simulink model "rx_chain_blockset"  (R2022b)
settings: Solver=VariableStepAuto  StartTime=0.0  StopTime=0  RelTol=1e-3
undefined symbols (not defined in the file or in its folder): rf, S
libraries: simrfV2elements x7, simrfV2util1 x4, rfBudgetAnalyzer_lib x3, simrfV2systems x2, simrfV2sources1 x1
settings Model: Creator=hessam  LastModifiedBy=hessam

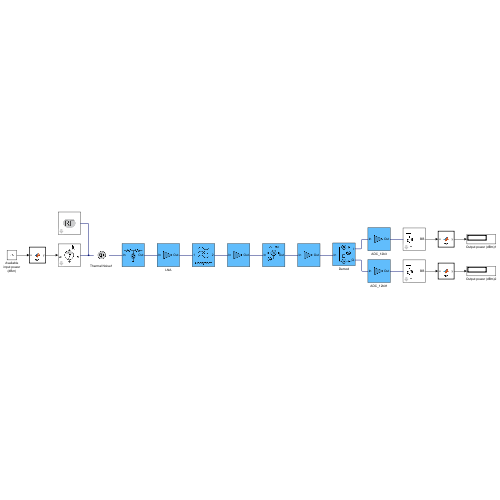
[thumbnail: Simulink's stored preview of the top-level diagram]
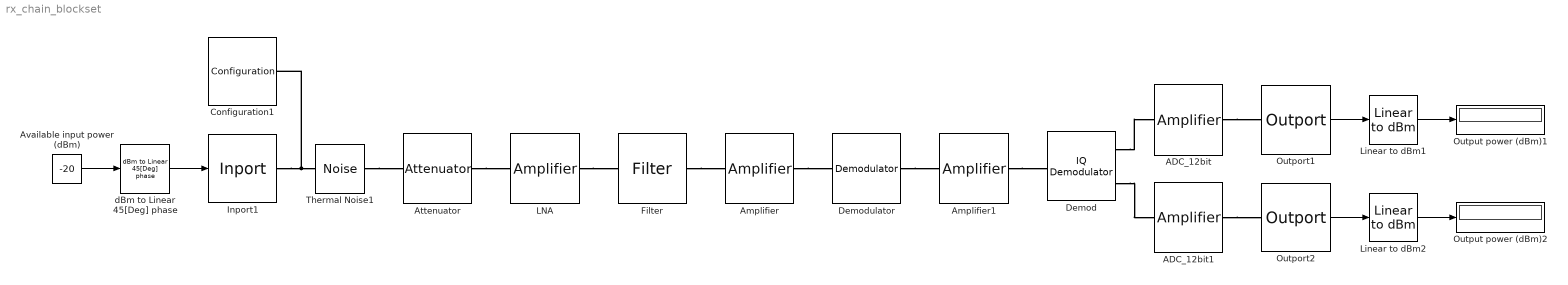
== system rx_chain_blockset ==
  ADC_12bit : simrfV2elements/Amplifier  classname=amplifier  DataSource=Data file  isNetworkObj=off  Paramtype=S-parameters  Sparam=[0 0;1 0]  SparamFreq=1e9 Hz  SparamZ0=50  isRationalObj=off  Residues=0  Poles=0  DF={0 0; 1 0}  Source_linear_gain=Available power gain  linear_gain=0 dB  AmAmAmPmTable=[-25,5,-1;-10,20,-2;0,27,5;5,28,12]  Zin=50  Zout=50  Source_Poly=Even and odd order  Poly_Coeffs=[0 1]  IPType=Output  IP2=Inf dBm  IP3=Inf dBm  P1dB=inf dBm  Psat=inf dBm  Gcomp=inf dBm  InternalGrounding=on  SourceFreq=Extracted from data source  PlotFreq=[1e9:1e6:3e9] Hz  PlotType=X-Y plane  YParam1=S(1,1)  YFormat1=Magnitude (dB)  YParam2=None  YFormat2=Magnitude (dB)  YOption=Linear  XOption=Linear  SparamRepresentation=Time domain (rationalfit)  FitTol=-40  FitOpt=Fit individually  MaxPoles=48  AutoImpulseLength=on  ImpulseLength=1e-10 s  MagModeling=off  AddNoise=on  NoiseType=Noise figure  NoiseDist=White  NF=25  MinNF=0  Gopt=0  RN=0  CarrierFreq=0 Hz  NoiseAutoImpulseLength=on  NoiseImpulseLength=1e-10 s  ConstS21NL=off  OpFreq=1 GHz  SetOpFreqAsMaxS21=off
  ADC_12bit1 : simrfV2elements/Amplifier  classname=amplifier  DataSource=Data file  isNetworkObj=off  Paramtype=S-parameters  Sparam=[0 0;1 0]  SparamFreq=1e9 Hz  SparamZ0=50  isRationalObj=off  Residues=0  Poles=0  DF={0 0; 1 0}  Source_linear_gain=Available power gain  linear_gain=0 dB  AmAmAmPmTable=[-25,5,-1;-10,20,-2;0,27,5;5,28,12]  Zin=50  Zout=50  Source_Poly=Even and odd order  Poly_Coeffs=[0 1]  IPType=Output  IP2=Inf dBm  IP3=Inf dBm  P1dB=inf dBm  Psat=inf dBm  Gcomp=inf dBm  InternalGrounding=on  SourceFreq=Extracted from data source  PlotFreq=[1e9:1e6:3e9] Hz  PlotType=X-Y plane  YParam1=S(1,1)  YFormat1=Magnitude (dB)  YParam2=None  YFormat2=Magnitude (dB)  YOption=Linear  XOption=Linear  SparamRepresentation=Time domain (rationalfit)  FitTol=-40  FitOpt=Fit individually  MaxPoles=48  AutoImpulseLength=on  ImpulseLength=1e-10 s  MagModeling=off  AddNoise=on  NoiseType=Noise figure  NoiseDist=White  NF=25  MinNF=0  Gopt=0  RN=0  CarrierFreq=0 Hz  NoiseAutoImpulseLength=on  NoiseImpulseLength=1e-10 s  ConstS21NL=off  OpFreq=1 GHz  SetOpFreqAsMaxS21=off
  Amplifier : simrfV2elements/Amplifier  classname=amplifier  DataSource=Data file  isNetworkObj=off  Paramtype=S-parameters  Sparam=[0 0;1 0]  SparamFreq=1e9 Hz  SparamZ0=50  isRationalObj=off  Residues=0  Poles=0  DF={0 0; 1 0}  Source_linear_gain=Available power gain  linear_gain=8 dB  AmAmAmPmTable=[-25,5,-1;-10,20,-2;0,27,5;5,28,12]  Zin=50  Zout=50  Source_Poly=Even and odd order  Poly_Coeffs=[0 1]  IPType=Output  IP2=Inf dBm  IP3=20 dBm  P1dB=inf dBm  Psat=inf dBm  Gcomp=inf dBm  InternalGrounding=on  SourceFreq=Extracted from data source  PlotFreq=[1e9:1e6:3e9] Hz  PlotType=X-Y plane  YParam1=S(1,1)  YFormat1=Magnitude (dB)  YParam2=None  YFormat2=Magnitude (dB)  YOption=Linear  XOption=Linear  SparamRepresentation=Time domain (rationalfit)  FitTol=-40  FitOpt=Fit individually  MaxPoles=48  AutoImpulseLength=on  ImpulseLength=1e-10 s  MagModeling=off  AddNoise=on  NoiseType=Noise figure  NoiseDist=White  NF=10  MinNF=0  Gopt=0  RN=0  CarrierFreq=0 Hz  NoiseAutoImpulseLength=on  NoiseImpulseLength=1e-10 s  ConstS21NL=off  OpFreq=1 GHz  SetOpFreqAsMaxS21=off
  Amplifier1 : simrfV2elements/Amplifier  classname=amplifier  DataSource=Data file  isNetworkObj=off  Paramtype=S-parameters  Sparam=[0 0;1 0]  SparamFreq=1e9 Hz  SparamZ0=50  isRationalObj=off  Residues=0  Poles=0  DF={0 0; 1 0}  Source_linear_gain=Available power gain  linear_gain=8 dB  AmAmAmPmTable=[-25,5,-1;-10,20,-2;0,27,5;5,28,12]  Zin=50  Zout=50  Source_Poly=Even and odd order  Poly_Coeffs=[0 1]  IPType=Output  IP2=Inf dBm  IP3=30 dBm  P1dB=inf dBm  Psat=inf dBm  Gcomp=inf dBm  InternalGrounding=on  SourceFreq=Extracted from data source  PlotFreq=[1e9:1e6:3e9] Hz  PlotType=X-Y plane  YParam1=S(1,1)  YFormat1=Magnitude (dB)  YParam2=None  YFormat2=Magnitude (dB)  YOption=Linear  XOption=Linear  SparamRepresentation=Time domain (rationalfit)  FitTol=-40  FitOpt=Fit individually  MaxPoles=48  AutoImpulseLength=on  ImpulseLength=1e-10 s  MagModeling=off  AddNoise=on  NoiseType=Noise figure  NoiseDist=White  NF=20  MinNF=0  Gopt=0  RN=0  CarrierFreq=0 Hz  NoiseAutoImpulseLength=on  NoiseImpulseLength=1e-10 s  ConstS21NL=off  OpFreq=1 GHz  SetOpFreqAsMaxS21=off
  Attenuator : simrfV2elements/Attenuator  classname=attenuator  Att=4  Zin=50  Zout=50  AddNoise=on  InternalGrounding=on
  Available input power (dBm) : Constant  Value=-20
  Configuration1 : simrfV2util1/Configuration  AutoFreq=on  Tones=[] Hz  Harmonics=[]  NormalizeCarrierPower=on  SolverType=Auto  UseCCode=on  StepSize=(1/116000000)/8 s  AddNoise=on  defaultRNG=on  Seed=0  Temperature=290.0 K  SolverDelFlag=0  AbsTol=1e-6  RelTol=1e-3  MaxIter=10  ErrorEstimationType=2-norm over all variables  EnableInterpFilter=on  HiddenFIRfilterControllerParam=off  SmallSignalApprox=off  AllSimFreqs=on  SimFreqs=[] Hz  SimFreqsInternal=[]  SamplesPerFrame=1
  Demod : simrfV2systems/IQ Demodulator  classname=iqdemod  Source_linear_gain=Available power gain  linear_gain=0 dB  Poly_Coeffs=[0 1]  LOFreq=11 GHz  Zin=50  Zout=50  AddIRFilter=off  AddCSFilters=on  InternalGrounding=on  ForceNextInit=off  Source_Poly=Even and odd order  IPType=Output  IP2=Inf dBm  IP3=30 dBm  P1dB=inf dBm  Psat=inf dBm  Gcomp=inf dBm  NF=20  GainMismatch=0 dB  PhaseMismatch=0 deg  Isolation=inf dB  AddPhaseNoise=off  PhaseNoiseOffset=1  PhaseNoiseLevel=-Inf  AutoImpulseLengthPN=on  ImpulseLengthPN=1e-10  ImpulseLength_unitPN=s  DesignMethodIR=Ideal  ResponseTypeIR=Highpass  ImplementationIR=LC Tee  ImplementationIdealIR=Constant per carrier  ImplementationRationalIR=Transfer function  UseFilterOrderIR=on  FilterOrderIR=3  PassFreq_lpIR=11.058  PassFreq_lp_unitIR=GHz  PassFreq_hpIR=10.942  PassFreq_hp_unitIR=GHz  PassFreq_bpIR=[10.942 11.058]  PassFreq_bp_unitIR=GHz  PassFreq_bsIR=[0 10.941999999]  PassFreq_bs_unitIR=GHz  PassAttenIR=10*log10(2)  StopFreq_lpIR=11.058000001  StopFreq_lp_unitIR=GHz  StopFreq_hpIR=10.941999999  StopFreq_hp_unitIR=GHz  StopFreq_bpIR=[10.941999999 11.058000001]  StopFreq_bp_unitIR=GHz  StopFreq_bsIR=[1e-09 10.942]  StopFreq_bs_unitIR=GHz  StopAttenIR=40  RsrcIR=50  RloadIR=50  AutoImpulseLengthIR=on  ImpulseLengthIR=1e-10  ImpulseLength_unitIR=s  DesignMethodCS=Ideal  ResponseTypeCS=Lowpass  ImplementationCS=LC Tee  ImplementationIdealCS=Constant per carrier  ImplementationRationalCS=Transfer function  UseFilterOrderCS=on  FilterOrderCS=3  PassFreq_lpCS=58  PassFreq_lp_unitCS=MHz  PassFreq_hpCS=0  PassFreq_hp_unitCS=Hz  PassFreq_bpCS=[0 58]  PassFreq_bp_unitCS=MHz  PassFreq_bsCS=[21.941999999 22.058000001]  PassFreq_bs_unitCS=GHz  PassAttenCS=10*log10(2)  StopFreq_lpCS=58.000001  StopFreq_lp_unitCS=MHz  StopFreq_hpCS=0  StopFreq_hp_unitCS=Hz  StopFreq_bpCS=[0 58.000001]  StopFreq_bp_unitCS=MHz  StopFreq_bsCS=[21.942 22.058]  StopFreq_bs_unitCS=GHz  StopAttenCS=40  RsrcCS=50  RloadCS=50  AutoImpulseLengthCS=on  ImpulseLengthCS=1e-10  ImpulseLength_unitCS=s
  Demodulator : simrfV2systems/Demodulator  classname=rfdemod  Source_linear_gain=Available power gain  linear_gain=-6 dB  Poly_Coeffs=[0 1]  LOFreq=66 GHz  Zin=50  Zout=50  AddIRFilter=on  AddCSFilter=on  InternalGrounding=on  ForceNextInit=off  Source_Poly=Even and odd order  IPType=Output  IP2=Inf dBm  IP3=25 dBm  P1dB=inf dBm  Psat=inf dBm  Gcomp=inf dBm  NF=15  Isolation=inf dB  AddPhaseNoise=off  PhaseNoiseOffset=1  PhaseNoiseLevel=-Inf  AutoImpulseLengthPN=on  ImpulseLengthPN=1e-10  ImpulseLength_unitPN=s  DesignMethodIR=Ideal  ResponseTypeIR=Highpass  ImplementationIR=LC Tee  ImplementationIdealIR=Constant per carrier  ImplementationRationalIR=Transfer function  UseFilterOrderIR=on  FilterOrderIR=3  PassFreq_lpIR=77.058  PassFreq_lp_unitIR=GHz  PassFreq_hpIR=76.942  PassFreq_hp_unitIR=GHz  PassFreq_bpIR=[76.942 77.058]  PassFreq_bp_unitIR=GHz  PassFreq_bsIR=[54.941999999 55.058000001]  PassFreq_bs_unitIR=GHz  PassAttenIR=10*log10(2)  StopFreq_lpIR=77.058000001  StopFreq_lp_unitIR=GHz  StopFreq_hpIR=76.941999999  StopFreq_hp_unitIR=GHz  StopFreq_bpIR=[76.941999999 77.058000001]  StopFreq_bp_unitIR=GHz  StopFreq_bsIR=[54.942 55.058]  StopFreq_bs_unitIR=GHz  StopAttenIR=40  RsrcIR=50  RloadIR=50  AutoImpulseLengthIR=on  ImpulseLengthIR=1e-10  ImpulseLength_unitIR=s  DesignMethodCS=Ideal  ResponseTypeCS=Lowpass  ImplementationCS=LC Tee  ImplementationIdealCS=Constant per carrier  ImplementationRationalCS=Transfer function  UseFilterOrderCS=on  FilterOrderCS=3  PassFreq_lpCS=11.058  PassFreq_lp_unitCS=GHz  PassFreq_hpCS=10.942  PassFreq_hp_unitCS=GHz  PassFreq_bpCS=[10.942 11.058]  PassFreq_bp_unitCS=GHz  PassFreq_bsCS=[142.941999999 143.058000001]  PassFreq_bs_unitCS=GHz  PassAttenCS=10*log10(2)  StopFreq_lpCS=11.058000001  StopFreq_lp_unitCS=GHz  StopFreq_hpCS=10.941999999  StopFreq_hp_unitCS=GHz  StopFreq_bpCS=[10.941999999 11.058000001]  StopFreq_bp_unitCS=GHz  StopFreq_bsCS=[142.942 143.058]  StopFreq_bs_unitCS=GHz  StopAttenCS=40  RsrcCS=50  RloadCS=50  AutoImpulseLengthCS=on  ImpulseLengthCS=1e-10  ImpulseLength_unitCS=s
  Filter : simrfV2elements/Filter  classname=filter  DesignMethod=Chebyshev  ResponseType=Bandstop  Implementation=LC Tee  ImplementationIdeal=Constant per carrier  ImplementationRational=Transfer function  UseFilterOrder=on  FilterOrder=3  PassFreq_lp=1 GHz  PassFreq_hp=2 GHz  PassFreq_bp=[2 3] GHz  PassFreq_bs=[1 4] GHz  PassAtten=3  StopFreq_lp=2 GHz  StopFreq_hp=1 GHz  StopFreq_bp=[1.5 3.5] GHz  StopFreq_bs=[50 60] GHz  StopAtten=40  Rsrc=50  Rload=50  AutoImpulseLength=on  ImpulseLength=1e-10 s  InternalGrounding=on  PlotFuncLeft=Voltage transfer  PlotLeftForm=Magnitude (dB)  PlotRightOnVT=None  PlotRightNoTD=None  PlotRightNoGD=None  PlotRightNoIR=None  PlotRightNoSR=None  PlotRightForm=Magnitude (dB)  FreqPoints=logspace(0,10,101)  Freq_unit=Hz  TimePoints=linspace(0,1,1e6+1)  Time_unit=s  XaxisScale=Linear  YaxisScale=Linear  needRedraw=0
  Inport1 : simrfV2util1/Inport  SimulinkInputSignalType=Power  CarrierFreq=77 GHz  ZS=50  UseSqWave=off  NumCoeff=10  Bias=0  DutyCyc=50  InternalGrounding=on
  LNA : simrfV2elements/Amplifier  classname=amplifier  DataSource=Data file  isNetworkObj=off  Paramtype=S-parameters  Sparam=[0 0;1 0]  SparamFreq=1e9 Hz  SparamZ0=50  isRationalObj=off  Residues=0  Poles=0  DF={0 0; 1 0}  Source_linear_gain=Available power gain  linear_gain=15 dB  AmAmAmPmTable=[-25,5,-1;-10,20,-2;0,27,5;5,28,12]  Zin=50  Zout=50  Source_Poly=Even and odd order  Poly_Coeffs=[0 1]  IPType=Output  IP2=Inf dBm  IP3=15 dBm  P1dB=inf dBm  Psat=inf dBm  Gcomp=inf dBm  InternalGrounding=on  SourceFreq=Extracted from data source  PlotFreq=[1e9:1e6:3e9] Hz  PlotType=X-Y plane  YParam1=S(1,1)  YFormat1=Magnitude (dB)  YParam2=None  YFormat2=Magnitude (dB)  YOption=Linear  XOption=Linear  SparamRepresentation=Time domain (rationalfit)  FitTol=-40  FitOpt=Fit individually  MaxPoles=48  AutoImpulseLength=on  ImpulseLength=1e-10 s  MagModeling=off  AddNoise=on  NoiseType=Noise figure  NoiseDist=White  NF=8  MinNF=0  Gopt=0  RN=0  CarrierFreq=0 Hz  NoiseAutoImpulseLength=on  NoiseImpulseLength=1e-10 s  ConstS21NL=off  OpFreq=1 GHz  SetOpFreqAsMaxS21=off
  Linear to dBm1 : rfBudgetAnalyzer_lib/Linear to dBm  SystemSampleTime=-1  VariantActivationTime=update diagram  Latency=0  AutoFrameSizeCalculation=off
  Linear to dBm2 : rfBudgetAnalyzer_lib/Linear to dBm  SystemSampleTime=-1  VariantActivationTime=update diagram  Latency=0  AutoFrameSizeCalculation=off
  Outport1 : simrfV2util1/Outport  SensorType=Power  OutputFormat=Complex Baseband  CarrierFreq=0 Hz  ZL=50  InternalGrounding=on  StepSize=1e-6 s  AutoStep=on
  Outport2 : simrfV2util1/Outport  SensorType=Power  OutputFormat=Complex Baseband  CarrierFreq=0 Hz  ZL=50  InternalGrounding=on  StepSize=1e-6 s  AutoStep=on
  Output power (dBm)1 : Display
  Output power (dBm)2 : Display
  Thermal Noise1 : simrfV2sources1/Noise  SimulinkInputSignalType=Ideal voltage  NoiseType=White  NoisePSD=4*rf.physconst('Boltzmann')*290*50  CarrierFreq=0 Hz  AutoImpulseLength=on  ImpulseLength=1e-10 s  InternalGrounding=off
  dBm to Linear 45[Deg] phase : rfBudgetAnalyzer_lib/dBm to Linear 45[Deg] phase  SystemSampleTime=-1  VariantActivationTime=update diagram  Latency=0  AutoFrameSizeCalculation=off
  wires:
  Available input power (dBm)/1 -> dBm to Linear 45[Deg] phase/1
  dBm to Linear 45[Deg] phase/1 -> Inport1/1
  Outport1/1 -> Linear to dBm1/1
  Outport2/1 -> Linear to dBm2/1
  Linear to dBm1/1 -> Output power (dBm)1/1
  Linear to dBm2/1 -> Output power (dBm)2/1
  connections:
  Configuration1/LConn1 -- Inport1/RConn1 -- Thermal Noise1/RConn1
  Thermal Noise1/LConn1 -- Attenuator/LConn1
  Attenuator/RConn1 -- LNA/LConn1
  LNA/RConn1 -- Filter/LConn1
  Filter/RConn1 -- Amplifier/LConn1
  Amplifier/RConn1 -- Demodulator/LConn1
  Demodulator/RConn1 -- Amplifier1/LConn1
  Amplifier1/RConn1 -- Demod/LConn1
  Demod/RConn1 -- ADC_12bit/LConn1
  Demod/RConn2 -- ADC_12bit1/LConn1
  ADC_12bit/RConn1 -- Outport1/LConn1
  ADC_12bit1/RConn1 -- Outport2/LConn1
